simulink model "untitled"  (R2018b)
settings: Solver=VariableStepAuto  StartTime=0.0  StopTime=10.0  RelTol=1e-3
libraries: neural x29
settings Model: Creator=Paweł Tymiński  LastModifiedBy=Paweł Tymiński

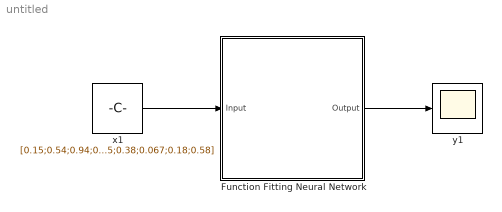
== system untitled ==
  Function Fitting Neural Network : Subsystem
      mask help: Function Fitting Neural Network
      mask Display: e = 0.06;c1 = [120 150 230]/255;c2 = ([120 150 230]+0)/383;c3 = ([120 150 230]+128)/383;patch([0 1 1 0],[0 0 1 1],c1);patch([0 1 1 1-e 1-e 0+e],[0 0 1 1-e 0+e 0+e],c2);patch([0 0 1 1-e 0+e 0+e],[0 1 1 1-e 1-e 0+e],c3);plot([0 1 1 0 0],[0 0 1 1 0]);fprintf('NNET');port_label('input',1,' Input');port_label('output',1,'Output ');
  x1 : Constant  Value=[0.15;0.54;0.94;0.66;0.39;0.26;0.85;0.95;0.38;0.067;0.18;0.58]  SampleTime=1
      mask Display: e = 0.06;c1 = [120 230 180]/255;c2 = ([120 230 180]+0)/(256+128);c3 = ([120 230 180]+128)/(256+128);patch([0 1 1 0],[0 0 1 1],c1);patch([0 1 1 1-e 1-e 0+e],[0 0 1 1-e 0+e 0+e],c2);patch([0 0 1 1-e 0+e 0+e],[0 1 1 1-e 1-e 0+e],c3);plot([0 1 1 0 0],[0 0 1 1 0]);disp('Constant');
  y1 : Scope
      mask Display: e = 0.06;c1 = [120 230 180]/255;c2 = ([120 230 180]+0)/(256+128);c3 = ([120 230 180]+128)/(256+128);patch([0 1 1 0],[0 0 1 1],c1);patch([0 1 1 1-e 1-e 0+e],[0 0 1 1-e 0+e 0+e],c2);patch([0 0 1 1-e 0+e 0+e],[0 1 1 1-e 1-e 0+e],c3);plot([0 1 1 0 0],[0 0 1 1 0]);plot([0.15 0.85 0.85 0.15 0.15],[0.5 0.5 0.85 0.85 0.5]);
  wires:
  x1/1 -> Function Fitting Neural Network/1(Input)
  Function Fitting Neural Network/1(Output) -> y1/1

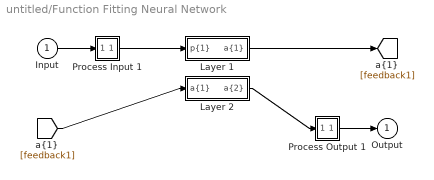
== system untitled/Function Fitting Neural Network ==
  Input : Inport  PortDimensions=12
      mask Display: e = 0.06;c1 = [120 230 180]/255;c2 = ([120 230 180]+0)/(256+128);c3 = ([120 230 180]+128)/(256+128);patch([0 1 1 0],[0 0 1 1],c1);patch([0 1 1 1-e 1-e 0+e],[0 0 1 1-e 0+e 0+e],c2);patch([0 0 1 1-e 0+e 0+e],[0 1 1 1-e 1-e 0+e],c3);plot([0 1 1 0 0],[0 0 1 1 0]);
  Layer 1 : Subsystem
      mask Display: e = 0.06;c1 = [120 150 230]/255;c2 = ([120 150 230]+0)/383;c3 = ([120 150 230]+128)/383;patch([0 1 1 0],[0 0 1 1],c1);patch([0 1 1 1-e 1-e 0+e],[0 0 1 1-e 0+e 0+e],c2);patch([0 0 1 1-e 0+e 0+e],[0 1 1 1-e 1-e 0+e],c3);plot([0 1 1 0 0],[0 0 1 1 0]);
  Layer 2 : Subsystem
      mask Display: e = 0.06;c1 = [120 150 230]/255;c2 = ([120 150 230]+0)/383;c3 = ([120 150 230]+128)/383;patch([0 1 1 0],[0 0 1 1],c1);patch([0 1 1 1-e 1-e 0+e],[0 0 1 1-e 0+e 0+e],c2);patch([0 0 1 1-e 0+e 0+e],[0 1 1 1-e 1-e 0+e],c3);plot([0 1 1 0 0],[0 0 1 1 0]);
  Process Input 1 : Subsystem
      mask Display: e = 0.06;c1 = [120 150 230]/255;c2 = ([120 150 230]+0)/383;c3 = ([120 150 230]+128)/383;patch([0 1 1 0],[0 0 1 1],c1);patch([0 1 1 1-e 1-e 0+e],[0 0 1 1-e 0+e 0+e],c2);patch([0 0 1 1-e 0+e 0+e],[0 1 1 1-e 1-e 0+e],c3);plot([0 1 1 0 0],[0 0 1 1 0]);
  Process Output 1 : Subsystem
      mask Display: e = 0.06;c1 = [120 150 230]/255;c2 = ([120 150 230]+0)/383;c3 = ([120 150 230]+128)/383;patch([0 1 1 0],[0 0 1 1],c1);patch([0 1 1 1-e 1-e 0+e],[0 0 1 1-e 0+e 0+e],c2);patch([0 0 1 1-e 0+e 0+e],[0 1 1 1-e 1-e 0+e],c3);plot([0 1 1 0 0],[0 0 1 1 0]);
  Output : Outport  InitialOutput=0
      mask Display: e = 0.06;c1 = [120 230 180]/255;c2 = ([120 230 180]+0)/(256+128);c3 = ([120 230 180]+128)/(256+128);patch([0 1 1 0],[0 0 1 1],c1);patch([0 1 1 1-e 1-e 0+e],[0 0 1 1-e 0+e 0+e],c2);patch([0 0 1 1-e 0+e 0+e],[0 1 1 1-e 1-e 0+e],c3);plot([0 1 1 0 0],[0 0 1 1 0]);
  wires:
  Input/1 -> Process Input 1/1(x)
  Process Output 1/1(y) -> Output/1
  Process Input 1/1(p) -> Layer 1/1("p{1}")
  Layer 1/1("a{1}") -> [feedback1]
  [feedback1] -> Layer 2/1("a{1} ")
  Layer 2/1("a{2}") -> Process Output 1/1(a)

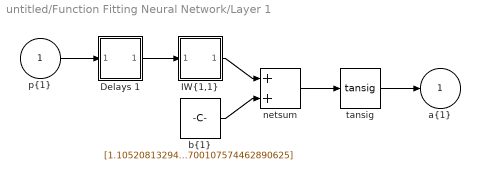
== system untitled/Function Fitting Neural Network/Layer 1 ==
  "p{1}" : Inport  PortDimensions=12
      mask Display: e = 0.06;c1 = [120 230 180]/255;c2 = ([120 230 180]+0)/(256+128);c3 = ([120 230 180]+128)/(256+128);patch([0 1 1 0],[0 0 1 1],c1);patch([0 1 1 1-e 1-e 0+e],[0 0 1 1-e 0+e 0+e],c2);patch([0 0 1 1-e 0+e 0+e],[0 1 1 1-e 1-e 0+e],c3);plot([0 1 1 0 0],[0 0 1 1 0]);
  Delays 1 : Subsystem
      mask Display: e = 0.06;c1 = [120 150 230]/255;c2 = ([120 150 230]+0)/383;c3 = ([120 150 230]+128)/383;patch([0 1 1 0],[0 0 1 1],c1);patch([0 1 1 1-e 1-e 0+e],[0 0 1 1-e 0+e 0+e],c2);patch([0 0 1 1-e 0+e 0+e],[0 1 1 1-e 1-e 0+e],c3);plot([0 1 1 0 0],[0 0 1 1 0]);disp('0');
  "IW{1,1}" : Subsystem
      mask Display: e = 0.06;c1 = [120 150 230]/255;c2 = ([120 150 230]+0)/383;c3 = ([120 150 230]+128)/383;patch([0 1 1 0],[0 0 1 1],c1);patch([0 1 1 1-e 1-e 0+e],[0 0 1 1-e 0+e 0+e],c2);patch([0 0 1 1-e 0+e 0+e],[0 1 1 1-e 1-e 0+e],c3);plot([0 1 1 0 0],[0 0 1 1 0]);disp('W');
  "b{1}" : Constant  Value=[1.105208132943532373104744692682288587093353271484375;0.396650909628887216040737939692917279899120330810546875;0.54239414591900725337580979612539522349834442138671875;0.2115757327206850835210616423864848911762237548828125;-0.4515141543103080579157904139719903469085693359375;0.61502574896100348222915954465861432254314422607421875;0.01756516716692051172099553468797239474952220916748046875;0.6012622440599362239055380996433086693286895751953125;-0.051598209526726834805998578303842805325984954833984375;0.1426075559304570139484980018096393905580043792724609375;-0.2304812660871213558788639375052298419177532196044921875;0.0678801928230618190074352469309815205633640289306640625;-0.1511582018231164281640843682907870970666408538818359375;-0.04926365002972421525129220754024572670459747314453125;0.108299861116097961843962593775358982384204864501953125;0.3436669062178363542869874436291866004467010498046875;-0.156260455829143996009378270173328928649425506591796875;0.69466705870215761375874308214406482875347137451171875;0.35182399411871634331561153885559178888797760009765625;1.013705487305092578509402301278896629810333251953125;-0.341177188449490298438604440889321267604827880859375;0.07182603963840873684265631027301424182951450347900390625;0.61566924743637507777549444654141552746295928955078125;-0.243279720160138490658852106207632459700107574462890625]
      mask Display: e = 0.06;c1 = [120 150 230]/255;c2 = ([120 150 230]+0)/383;c3 = ([120 150 230]+128)/383;patch([0 1 1 0],[0 0 1 1],c1);patch([0 1 1 1-e 1-e 0+e],[0 0 1 1-e 0+e 0+e],c2);patch([0 0 1 1-e 0+e 0+e],[0 1 1 1-e 1-e 0+e],c3);plot([0 1 1 0 0],[0 0 1 1 0]);disp('b');
  netsum : Sum  Inputs=2  SaturateOnIntegerOverflow=on  InputSameDT=on  OutDataTypeStr=Inherit: Same as first input
      mask Display: e = 0.06;c1 = [120 150 230]/255;c2 = ([120 150 230]+0)/383;c3 = ([120 150 230]+128)/383;patch([0 1 1 0],[0 0 1 1],c1);patch([0 1 1 1-e 1-e 0+e],[0 0 1 1-e 0+e 0+e],c2);patch([0 0 1 1-e 0+e 0+e],[0 1 1 1-e 1-e 0+e],c3);plot([0 1 1 0 0],[0 0 1 1 0]);disp('+');
  tansig : neural/Transfer Functions/tansig
  "a{1}" : Outport  InitialOutput=[0;0;0;0;0;0;0;0;0;0;0;0;0;0;0;0;0;0;0;0;0;0;0;0]
      mask Display: e = 0.06;c1 = [120 230 180]/255;c2 = ([120 230 180]+0)/(256+128);c3 = ([120 230 180]+128)/(256+128);patch([0 1 1 0],[0 0 1 1],c1);patch([0 1 1 1-e 1-e 0+e],[0 0 1 1-e 0+e 0+e],c2);patch([0 0 1 1-e 0+e 0+e],[0 1 1 1-e 1-e 0+e],c3);plot([0 1 1 0 0],[0 0 1 1 0]);
  wires:
  "p{1}"/1 -> Delays 1/1("p{1}")
  Delays 1/1("pd{1,1}") -> "IW{1,1}"/1("pd{1,1}")
  "IW{1,1}"/1("iz{1,1}") -> netsum/1
  "b{1}"/1 -> netsum/2
  netsum/1 -> tansig/1
  tansig/1 -> "a{1}"/1

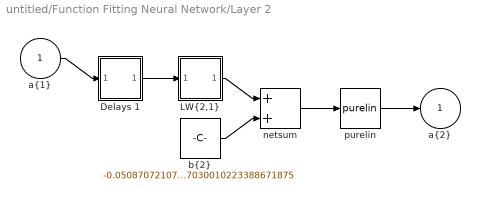
== system untitled/Function Fitting Neural Network/Layer 2 ==
  "a{1} " : Inport  PortDimensions=24
      mask Display: e = 0.06;c1 = [120 230 180]/255;c2 = ([120 230 180]+0)/(256+128);c3 = ([120 230 180]+128)/(256+128);patch([0 1 1 0],[0 0 1 1],c1);patch([0 1 1 1-e 1-e 0+e],[0 0 1 1-e 0+e 0+e],c2);patch([0 0 1 1-e 0+e 0+e],[0 1 1 1-e 1-e 0+e],c3);plot([0 1 1 0 0],[0 0 1 1 0]);
  Delays 1 : Subsystem
      mask Display: e = 0.06;c1 = [120 150 230]/255;c2 = ([120 150 230]+0)/383;c3 = ([120 150 230]+128)/383;patch([0 1 1 0],[0 0 1 1],c1);patch([0 1 1 1-e 1-e 0+e],[0 0 1 1-e 0+e 0+e],c2);patch([0 0 1 1-e 0+e 0+e],[0 1 1 1-e 1-e 0+e],c3);plot([0 1 1 0 0],[0 0 1 1 0]);disp('0');
  "LW{2,1}" : Subsystem
      mask Display: e = 0.06;c1 = [120 150 230]/255;c2 = ([120 150 230]+0)/383;c3 = ([120 150 230]+128)/383;patch([0 1 1 0],[0 0 1 1],c1);patch([0 1 1 1-e 1-e 0+e],[0 0 1 1-e 0+e 0+e],c2);patch([0 0 1 1-e 0+e 0+e],[0 1 1 1-e 1-e 0+e],c3);plot([0 1 1 0 0],[0 0 1 1 0]);disp('W');
  "b{2}" : Constant  Value=-0.050870721070801087904111881243807147257030010223388671875
      mask Display: e = 0.06;c1 = [120 150 230]/255;c2 = ([120 150 230]+0)/383;c3 = ([120 150 230]+128)/383;patch([0 1 1 0],[0 0 1 1],c1);patch([0 1 1 1-e 1-e 0+e],[0 0 1 1-e 0+e 0+e],c2);patch([0 0 1 1-e 0+e 0+e],[0 1 1 1-e 1-e 0+e],c3);plot([0 1 1 0 0],[0 0 1 1 0]);disp('b');
  netsum : Sum  Inputs=2  SaturateOnIntegerOverflow=on  InputSameDT=on  OutDataTypeStr=Inherit: Same as first input
      mask Display: e = 0.06;c1 = [120 150 230]/255;c2 = ([120 150 230]+0)/383;c3 = ([120 150 230]+128)/383;patch([0 1 1 0],[0 0 1 1],c1);patch([0 1 1 1-e 1-e 0+e],[0 0 1 1-e 0+e 0+e],c2);patch([0 0 1 1-e 0+e 0+e],[0 1 1 1-e 1-e 0+e],c3);plot([0 1 1 0 0],[0 0 1 1 0]);disp('+');
  purelin : neural/Transfer Functions/purelin
  "a{2}" : Outport  InitialOutput=0
      mask Display: e = 0.06;c1 = [120 230 180]/255;c2 = ([120 230 180]+0)/(256+128);c3 = ([120 230 180]+128)/(256+128);patch([0 1 1 0],[0 0 1 1],c1);patch([0 1 1 1-e 1-e 0+e],[0 0 1 1-e 0+e 0+e],c2);patch([0 0 1 1-e 0+e 0+e],[0 1 1 1-e 1-e 0+e],c3);plot([0 1 1 0 0],[0 0 1 1 0]);
  wires:
  "a{1} "/1 -> Delays 1/1("p{2}")
  Delays 1/1("pd{2,1}") -> "LW{2,1}"/1("ad{2,1}")
  "LW{2,1}"/1("lz{2,1}") -> netsum/1
  "b{2}"/1 -> netsum/2
  netsum/1 -> purelin/1
  purelin/1 -> "a{2}"/1

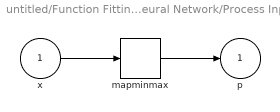
== system untitled/Function Fitting Neural Network/Process Input 1 ==
  x : Inport  PortDimensions=12
      mask Display: e = 0.06;c1 = [120 230 180]/255;c2 = ([120 230 180]+0)/(256+128);c3 = ([120 230 180]+128)/(256+128);patch([0 1 1 0],[0 0 1 1],c1);patch([0 1 1 1-e 1-e 0+e],[0 0 1 1-e 0+e 0+e],c2);patch([0 0 1 1-e 0+e 0+e],[0 1 1 1-e 1-e 0+e],c3);plot([0 1 1 0 0],[0 0 1 1 0]);
  mapminmax : neural/Processing Functions/mapminmax  xmin=[-3.14159265358979311599796346854;-3.14159265358979311599796346854;-3.14159265358979311599796346854;-3.14159265358979311599796346854;-3.14159265358979311599796346854;-3.14159265358979311599796346854;-3.14159265358979311599796346854;-3.14159265358979311599796346854;-3.14159265358979311599796346854;-3.14159265358979311599796346854;-3.14159265358979311599796346854;-3.14159265358979311599796346854]  xmax=[3.14159265358979311599796346854;3.14159265358979311599796346854;3.14159265358979311599796346854;3.14159265358979311599796346854;3.14159265358979311599796346854;3.14159265358979311599796346854;3.14159265358979311599796346854;3.14159265358979311599796346854;3.14159265358979311599796346854;3.14159265358979311599796346854;3.14159265358979311599796346854;3.14159265358979311599796346854]  ymin=-1  ymax=1
  p : Outport  PortDimensions=12
      mask Display: e = 0.06;c1 = [120 230 180]/255;c2 = ([120 230 180]+0)/(256+128);c3 = ([120 230 180]+128)/(256+128);patch([0 1 1 0],[0 0 1 1],c1);patch([0 1 1 1-e 1-e 0+e],[0 0 1 1-e 0+e 0+e],c2);patch([0 0 1 1-e 0+e 0+e],[0 1 1 1-e 1-e 0+e],c3);plot([0 1 1 0 0],[0 0 1 1 0]);
  wires:
  x/1 -> mapminmax/1
  mapminmax/1 -> p/1

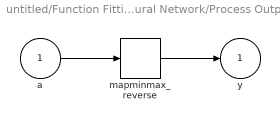
== system untitled/Function Fitting Neural Network/Process Output 1 ==
  a : Inport  PortDimensions=1
      mask Display: e = 0.06;c1 = [120 230 180]/255;c2 = ([120 230 180]+0)/(256+128);c3 = ([120 230 180]+128)/(256+128);patch([0 1 1 0],[0 0 1 1],c1);patch([0 1 1 1-e 1-e 0+e],[0 0 1 1-e 0+e 0+e],c2);patch([0 0 1 1-e 0+e 0+e],[0 1 1 1-e 1-e 0+e],c3);plot([0 1 1 0 0],[0 0 1 1 0]);
  mapminmax_reverse : neural/Processing Functions/mapminmax_reverse  xmin=-0.246707831183186704349097340128  xmax=0.224645518642549779642081375641  ymin=-1  ymax=1
  y : Outport  PortDimensions=1
      mask Display: e = 0.06;c1 = [120 230 180]/255;c2 = ([120 230 180]+0)/(256+128);c3 = ([120 230 180]+128)/(256+128);patch([0 1 1 0],[0 0 1 1],c1);patch([0 1 1 1-e 1-e 0+e],[0 0 1 1-e 0+e 0+e],c2);patch([0 0 1 1-e 0+e 0+e],[0 1 1 1-e 1-e 0+e],c3);plot([0 1 1 0 0],[0 0 1 1 0]);
  wires:
  a/1 -> mapminmax_reverse/1
  mapminmax_reverse/1 -> y/1

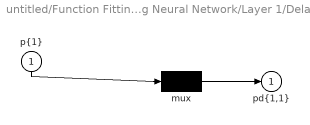
== system untitled/Function Fitting Neural Network/Layer 1/Delays 1 ==
  "p{1}" : Inport  PortDimensions=12
      mask Display: e = 0.06;c1 = [120 230 180]/255;c2 = ([120 230 180]+0)/(256+128);c3 = ([120 230 180]+128)/(256+128);patch([0 1 1 0],[0 0 1 1],c1);patch([0 1 1 1-e 1-e 0+e],[0 0 1 1-e 0+e 0+e],c2);patch([0 0 1 1-e 0+e 0+e],[0 1 1 1-e 1-e 0+e],c3);plot([0 1 1 0 0],[0 0 1 1 0]);
  mux : Mux  Inputs=1
      mask Display: e = 0.06;c1 = [120 150 230]/255;c2 = ([120 150 230]+0)/383;c3 = ([120 150 230]+128)/383;patch([0 1 1 0],[0 0 1 1],c1);patch([0 1 1 1-e 1-e 0+e],[0 0 1 1-e 0+e 0+e],c2);patch([0 0 1 1-e 0+e 0+e],[0 1 1 1-e 1-e 0+e],c3);plot([0 1 1 0 0],[0 0 1 1 0]);disp('Mux')
  "pd{1,1}" : Outport
      mask Display: e = 0.06;c1 = [120 230 180]/255;c2 = ([120 230 180]+0)/(256+128);c3 = ([120 230 180]+128)/(256+128);patch([0 1 1 0],[0 0 1 1],c1);patch([0 1 1 1-e 1-e 0+e],[0 0 1 1-e 0+e 0+e],c2);patch([0 0 1 1-e 0+e 0+e],[0 1 1 1-e 1-e 0+e],c3);plot([0 1 1 0 0],[0 0 1 1 0]);
  wires:
  "p{1}"/1 -> mux/1
  mux/1 -> "pd{1,1}"/1

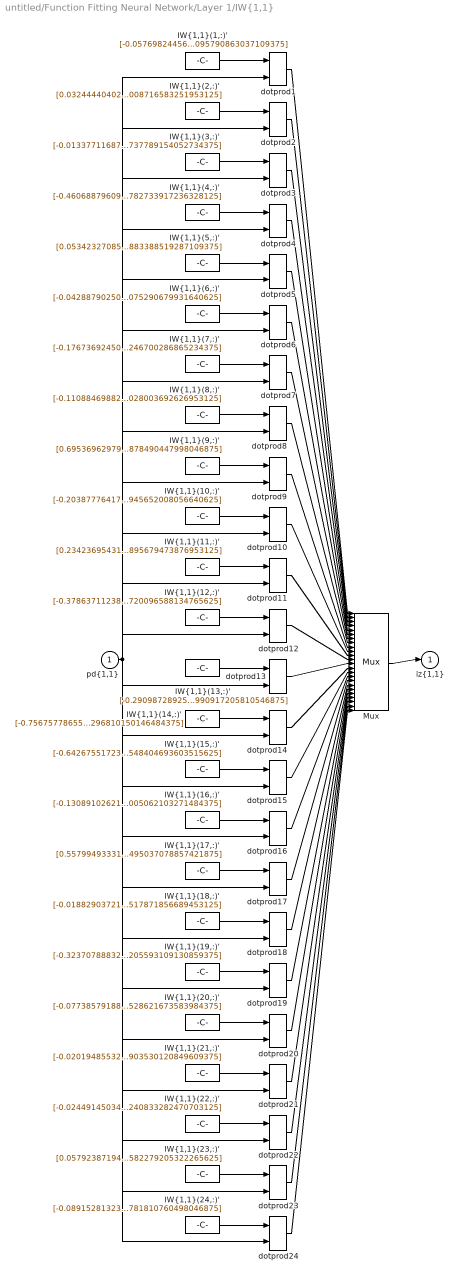
== system untitled/Function Fitting Neural Network/Layer 1/IW{1,1} ==
  "pd{1,1}" : Inport  PortDimensions=12
      mask Display: e = 0.06;c1 = [120 230 180]/255;c2 = ([120 230 180]+0)/(256+128);c3 = ([120 230 180]+128)/(256+128);patch([0 1 1 0],[0 0 1 1],c1);patch([0 1 1 1-e 1-e 0+e],[0 0 1 1-e 0+e 0+e],c2);patch([0 0 1 1-e 0+e 0+e],[0 1 1 1-e 1-e 0+e],c3);plot([0 1 1 0 0],[0 0 1 1 0]);
  "IW{1,1}(1,:)'" : Constant  Value=[-0.0576982445657482634349122463390813209116458892822265625;0.109430497477228716451946866072830744087696075439453125;-0.057052816673429408711459842606927850283682346343994140625;-0.00556308798543494499588835111580920056439936161041259765625;-0.6259020264135053412957176988129504024982452392578125;0.016003567569307701468073190653740311972796916961669921875;-0.8434917592845418976565952107193879783153533935546875;-0.82946259040420156072315194251132197678089141845703125;0.1764068613029800836056182333777542226016521453857421875;0.145967761274977736452029830616083927452564239501953125;-0.058731224497028937381326585409624385647475719451904296875;-0.81088898160597400188720484948134981095790863037109375]
      mask Display: e = 0.06;c1 = [120 150 230]/255;c2 = ([120 150 230]+0)/383;c3 = ([120 150 230]+128)/383;patch([0 1 1 0],[0 0 1 1],c1);patch([0 1 1 1-e 1-e 0+e],[0 0 1 1-e 0+e 0+e],c2);patch([0 0 1 1-e 0+e 0+e],[0 1 1 1-e 1-e 0+e],c3);plot([0 1 1 0 0],[0 0 1 1 0]);disp('Weights');
  "IW{1,1}(10,:)'" : Constant  Value=[-0.2038777641723933109485500381197198294103145599365234375;-0.09127744128260480149794631188342464156448841094970703125;-0.250425668125327349766706674927263520658016204833984375;-0.6005356078893466786894350661896169185638427734375;0.463817738348928643166146912335534580051898956298828125;-0.22254593099828123836658733125659637153148651123046875;0.58826545020638132399426467600278556346893310546875;0.44769782814802205894721964796190150082111358642578125;-0.62152830059035946153045415485394187271595001220703125;0.002081110896482388054884449246628719265572726726531982421875;-0.1693741871775031049285331619103089906275272369384765625;0.432919576819769391651249179631122387945652008056640625]
      mask Display: e = 0.06;c1 = [120 150 230]/255;c2 = ([120 150 230]+0)/383;c3 = ([120 150 230]+128)/383;patch([0 1 1 0],[0 0 1 1],c1);patch([0 1 1 1-e 1-e 0+e],[0 0 1 1-e 0+e 0+e],c2);patch([0 0 1 1-e 0+e 0+e],[0 1 1 1-e 1-e 0+e],c3);plot([0 1 1 0 0],[0 0 1 1 0]);disp('Weights');
  "IW{1,1}(11,:)'" : Constant  Value=[0.234236954316088319405508855197695083916187286376953125;-0.18360567694735241417447468847967684268951416015625;0.29527725169132512661462897085584700107574462890625;-0.07852522350352102165071954686936805956065654754638671875;-0.02499587978778217145503504070802591741085052490234375;0.55075537422061227044167708299937658011913299560546875;0.404000823445536727529514564594137482345104217529296875;0.44417301193162372907607959859888069331645965576171875;-0.098084331859639439787912351675913669168949127197265625;0.1552805895459416218873371917652548290789127349853515625;-0.105223174288441023715989786069258116185665130615234375;0.0273825467705861858025429000917938537895679473876953125]
      mask Display: e = 0.06;c1 = [120 150 230]/255;c2 = ([120 150 230]+0)/383;c3 = ([120 150 230]+128)/383;patch([0 1 1 0],[0 0 1 1],c1);patch([0 1 1 1-e 1-e 0+e],[0 0 1 1-e 0+e 0+e],c2);patch([0 0 1 1-e 0+e 0+e],[0 1 1 1-e 1-e 0+e],c3);plot([0 1 1 0 0],[0 0 1 1 0]);disp('Weights');
  "IW{1,1}(12,:)'" : Constant  Value=[-0.378637112386513818851341284243972040712833404541015625;0.037594262190869316697661162152144243009388446807861328125;-0.34276628323199143100197261446737684309482574462890625;0.5610059674731131540426076753647066652774810791015625;-0.234742924109086203987573071572114713490009307861328125;-0.34498433455168420191938594143721275031566619873046875;-0.40093355732895552545613782058353535830974578857421875;-0.244379228588640196040415730749373324215412139892578125;-0.2081185533989977354263345432627829723060131072998046875;-0.303788026176015024670817865626304410398006439208984375;0.497969472273695590303077551652677357196807861328125;-0.1530896961062103989181792940144077874720096588134765625]
      mask Display: e = 0.06;c1 = [120 150 230]/255;c2 = ([120 150 230]+0)/383;c3 = ([120 150 230]+128)/383;patch([0 1 1 0],[0 0 1 1],c1);patch([0 1 1 1-e 1-e 0+e],[0 0 1 1-e 0+e 0+e],c2);patch([0 0 1 1-e 0+e 0+e],[0 1 1 1-e 1-e 0+e],c3);plot([0 1 1 0 0],[0 0 1 1 0]);disp('Weights');
  "IW{1,1}(13,:)'" : Constant  Value=[-0.29098728925777483933501343926764093339443206787109375;-0.23403889436192637507616609582328237593173980712890625;-0.32648452880923806151969301936333067715167999267578125;0.37033303451168120279390905125183053314685821533203125;0.35741048081226012289590698856045491993427276611328125;-0.450714597452358589624310525323380716145038604736328125;-0.3935563897871983130016815266571938991546630859375;-0.169607468869786448539827006243285723030567169189453125;0.03627189488180206089484869380612508393824100494384765625;-0.255262783153725136831013742266804911196231842041015625;0.5406240190514794985432445173501037061214447021484375;0.3912157641259550455714588679256848990917205810546875]
      mask Display: e = 0.06;c1 = [120 150 230]/255;c2 = ([120 150 230]+0)/383;c3 = ([120 150 230]+128)/383;patch([0 1 1 0],[0 0 1 1],c1);patch([0 1 1 1-e 1-e 0+e],[0 0 1 1-e 0+e 0+e],c2);patch([0 0 1 1-e 0+e 0+e],[0 1 1 1-e 1-e 0+e],c3);plot([0 1 1 0 0],[0 0 1 1 0]);disp('Weights');
  "IW{1,1}(14,:)'" : Constant  Value=[-0.75675778655779823989036003695218823850154876708984375;-0.57256728570934745103926388765103183686733245849609375;-0.69813783058899481215320292903925292193889617919921875;0.341299029411496090968825001255027018487453460693359375;0.251303173023257497842308794133714400231838226318359375;-0.404678403021913657422459209556109271943569183349609375;-0.46178764454366716396549463752307929098606109619140625;-0.612694179813959127756106681772507727146148681640625;-0.1787251079729085534442134530763723887503147125244140625;-0.0708295086322307809734155625847051851451396942138671875;0.28467844523556140590159202474751509726047515869140625;0.253402445405866261207705747438012622296810150146484375]
      mask Display: e = 0.06;c1 = [120 150 230]/255;c2 = ([120 150 230]+0)/383;c3 = ([120 150 230]+128)/383;patch([0 1 1 0],[0 0 1 1],c1);patch([0 1 1 1-e 1-e 0+e],[0 0 1 1-e 0+e 0+e],c2);patch([0 0 1 1-e 0+e 0+e],[0 1 1 1-e 1-e 0+e],c3);plot([0 1 1 0 0],[0 0 1 1 0]);disp('Weights');
  "IW{1,1}(15,:)'" : Constant  Value=[-0.642675517239493121479654291761107742786407470703125;0.454770625971706754508971926043159328401088714599609375;-0.55909130185978284099945767593453638255596160888671875;-0.324232449901053210172818808132433332502841949462890625;-0.3021864416171464728932960497331805527210235595703125;0.025746204309359012329938565244447090663015842437744140625;0.29076344251290031639456401535426266491413116455078125;0.287224819587555690869606905835098586976528167724609375;0.5660394222826548027427406850620172917842864990234375;0.59714965990429702547004353618831373751163482666015625;0.1381454207647970500172363017554744146764278411865234375;-0.1817547750427616348734005669030011631548404693603515625]
      mask Display: e = 0.06;c1 = [120 150 230]/255;c2 = ([120 150 230]+0)/383;c3 = ([120 150 230]+128)/383;patch([0 1 1 0],[0 0 1 1],c1);patch([0 1 1 1-e 1-e 0+e],[0 0 1 1-e 0+e 0+e],c2);patch([0 0 1 1-e 0+e 0+e],[0 1 1 1-e 1-e 0+e],c3);plot([0 1 1 0 0],[0 0 1 1 0]);disp('Weights');
  "IW{1,1}(16,:)'" : Constant  Value=[-0.130891026211613858976079427520744502544403076171875;0.66844103513181496456496688551851548254489898681640625;-0.077856732269279138591855371487326920032501220703125;-0.232472090221449156910438205159152857959270477294921875;-0.255710980073264926293319376782164908945560455322265625;-0.4776360697880968064765738745336420834064483642578125;-0.43032739202462166883123018124024383723735809326171875;-0.315093839860602853431004177764407359063625335693359375;0.42425139290134550318356332354596816003322601318359375;0.1627815184339168330662772632422274909913539886474609375;-0.175561382573102442439250125971739180386066436767578125;-0.195398308804458353815647342344163917005062103271484375]
      mask Display: e = 0.06;c1 = [120 150 230]/255;c2 = ([120 150 230]+0)/383;c3 = ([120 150 230]+128)/383;patch([0 1 1 0],[0 0 1 1],c1);patch([0 1 1 1-e 1-e 0+e],[0 0 1 1-e 0+e 0+e],c2);patch([0 0 1 1-e 0+e 0+e],[0 1 1 1-e 1-e 0+e],c3);plot([0 1 1 0 0],[0 0 1 1 0]);disp('Weights');
  "IW{1,1}(17,:)'" : Constant  Value=[0.55799493331606042634263076251954771578311920166015625;-0.22309655693261698505835965988808311522006988525390625;0.6126227320923636199268003110773861408233642578125;0.58402488695494059189883273575105704367160797119140625;0.0611459190998968338259800248124520294368267059326171875;-0.1009568503039272313603902375689358450472354888916015625;-0.0027857496668865773352397052775586416828446090221405029296875;-0.043533707626254448952440867515178979374468326568603515625;-0.423914476654462302196435530277085490524768829345703125;-0.297306405257678652009900588382151909172534942626953125;0.31034488341500965358221719725406728684902191162109375;0.138219760650011458391617225061054341495037078857421875]
      mask Display: e = 0.06;c1 = [120 150 230]/255;c2 = ([120 150 230]+0)/383;c3 = ([120 150 230]+128)/383;patch([0 1 1 0],[0 0 1 1],c1);patch([0 1 1 1-e 1-e 0+e],[0 0 1 1-e 0+e 0+e],c2);patch([0 0 1 1-e 0+e 0+e],[0 1 1 1-e 1-e 0+e],c3);plot([0 1 1 0 0],[0 0 1 1 0]);disp('Weights');
  "IW{1,1}(18,:)'" : Constant  Value=[-0.0188290372159080586500490284151965170167386531829833984375;0.08571894067923425952759686197168775834143161773681640625;0.07476998276994810399553870183808612637221813201904296875;-0.26273279809814109597709830268286168575286865234375;0.74529773641065133471528270092676393687725067138671875;0.2287956900511584346080695695491158403456211090087890625;0.100676777302572684202885966442408971488475799560546875;0.10545777470751178939156744718275149352848529815673828125;-0.33779422396237623882342404613154940307140350341796875;-0.10004153793748025991217076580142020247876644134521484375;-0.314650660060184328425947342111612670123577117919921875;0.717674975622703659183798663434572517871856689453125]
      mask Display: e = 0.06;c1 = [120 150 230]/255;c2 = ([120 150 230]+0)/383;c3 = ([120 150 230]+128)/383;patch([0 1 1 0],[0 0 1 1],c1);patch([0 1 1 1-e 1-e 0+e],[0 0 1 1-e 0+e 0+e],c2);patch([0 0 1 1-e 0+e 0+e],[0 1 1 1-e 1-e 0+e],c3);plot([0 1 1 0 0],[0 0 1 1 0]);disp('Weights');
  "IW{1,1}(19,:)'" : Constant  Value=[-0.323707888322097014910383450114750303328037261962890625;-0.1829168855639349555719519457852584309875965118408203125;-0.330005694199064947280675141882966272532939910888671875;-0.731949829581310940085359106888063251972198486328125;-0.08612571232734229920158242066463571973145008087158203125;-0.08059809728553703200848445931114838458597660064697265625;-0.87760323631197678651005844585597515106201171875;-0.80758494986182449704159580505802296102046966552734375;-0.60381485601594520051804693139274604618549346923828125;-0.094564858083827363355311490522581152617931365966796875;-0.1287633543330141960847612381257931701838970184326171875;-0.184875298135876331429017227492295205593109130859375]
      mask Display: e = 0.06;c1 = [120 150 230]/255;c2 = ([120 150 230]+0)/383;c3 = ([120 150 230]+128)/383;patch([0 1 1 0],[0 0 1 1],c1);patch([0 1 1 1-e 1-e 0+e],[0 0 1 1-e 0+e 0+e],c2);patch([0 0 1 1-e 0+e 0+e],[0 1 1 1-e 1-e 0+e],c3);plot([0 1 1 0 0],[0 0 1 1 0]);disp('Weights');
  "IW{1,1}(2,:)'" : Constant  Value=[0.032444404023012941851167312279358156956732273101806640625;0.04414553061315297510791566537591279484331607818603515625;-0.0106112782487167885137058220834660460241138935089111328125;-0.048784886253699526192928459522590856067836284637451171875;0.2277580941245788415105977264829562045633792877197265625;-0.033054502953275687049394804262192337773740291595458984375;-0.227154873776603649648819782669306732714176177978515625;-0.280258960188446260008987565015559084713459014892578125;0.042431749134326561534447108670065063051879405975341796875;0.02391057263545350031197500584312365390360355377197265625;0.56944118083220163217816889300593174993991851806640625;0.228972666740030750265333381321397610008716583251953125]
      mask Display: e = 0.06;c1 = [120 150 230]/255;c2 = ([120 150 230]+0)/383;c3 = ([120 150 230]+128)/383;patch([0 1 1 0],[0 0 1 1],c1);patch([0 1 1 1-e 1-e 0+e],[0 0 1 1-e 0+e 0+e],c2);patch([0 0 1 1-e 0+e 0+e],[0 1 1 1-e 1-e 0+e],c3);plot([0 1 1 0 0],[0 0 1 1 0]);disp('Weights');
  "IW{1,1}(20,:)'" : Constant  Value=[-0.077385791888315680342458335871924646198749542236328125;-0.07791169269795907015296876352294930256903171539306640625;-0.1197486847395914655312054719615844078361988067626953125;0.01236999838006685135949336284966193488799035549163818359375;-0.12042939319783500795590924781208741478621959686279296875;0.1777993058522819025402128545465529896318912506103515625;1.256154726931602905182217000401578843593597412109375;1.1044308939133369307228349498473107814788818359375;-0.06957830754075521040302731989868334494531154632568359375;0.06102650058959908918598813443168182857334613800048828125;0.1265492084764261171425658858424867503345012664794921875;-0.12455408350473749778952736733117490075528621673583984375]
      mask Display: e = 0.06;c1 = [120 150 230]/255;c2 = ([120 150 230]+0)/383;c3 = ([120 150 230]+128)/383;patch([0 1 1 0],[0 0 1 1],c1);patch([0 1 1 1-e 1-e 0+e],[0 0 1 1-e 0+e 0+e],c2);patch([0 0 1 1-e 0+e 0+e],[0 1 1 1-e 1-e 0+e],c3);plot([0 1 1 0 0],[0 0 1 1 0]);disp('Weights');
  "IW{1,1}(21,:)'" : Constant  Value=[-0.0201948553262207806946459953678640886209905147552490234375;-0.23862416360800586812018764248932711780071258544921875;-0.0624075719155085806288951744136284105479717254638671875;-0.2050412304881187586236279685181216336786746978759765625;0.57755863849575195256846882330137304961681365966796875;-0.1868015885482841864639880213871947489678859710693359375;-1.1297969667168483720587346397223882377147674560546875;-1.0499418410353704711468481036718003451824188232421875;0.11028483750953076147904852177816792391240596771240234375;-0.01477289766724391821550721459743726882152259349822998046875;-0.36103070488242094970843254486680962145328521728515625;0.490549489427872520419526836121804080903530120849609375]
      mask Display: e = 0.06;c1 = [120 150 230]/255;c2 = ([120 150 230]+0)/383;c3 = ([120 150 230]+128)/383;patch([0 1 1 0],[0 0 1 1],c1);patch([0 1 1 1-e 1-e 0+e],[0 0 1 1-e 0+e 0+e],c2);patch([0 0 1 1-e 0+e 0+e],[0 1 1 1-e 1-e 0+e],c3);plot([0 1 1 0 0],[0 0 1 1 0]);disp('Weights');
  "IW{1,1}(22,:)'" : Constant  Value=[-0.0244914503415263780372601587487224605865776538848876953125;-0.364372965754643729496820014901459217071533203125;0.0243159411388128264552843660339931375347077846527099609375;-0.37098362235615400805954777752049267292022705078125;-0.4495515370744975758299233348225243389606475830078125;-0.136068426983480039726970289848395623266696929931640625;0.93762933653948088430496454748208634555339813232421875;0.90477946186466839950668372694053687155246734619140625;-0.03000179655139802170626950328369275666773319244384765625;-0.02314507042774012479657841367952642031013965606689453125;-0.3708231204690406457302742637693881988525390625;-0.459923018655834792145498113313806243240833282470703125]
      mask Display: e = 0.06;c1 = [120 150 230]/255;c2 = ([120 150 230]+0)/383;c3 = ([120 150 230]+128)/383;patch([0 1 1 0],[0 0 1 1],c1);patch([0 1 1 1-e 1-e 0+e],[0 0 1 1-e 0+e 0+e],c2);patch([0 0 1 1-e 0+e 0+e],[0 1 1 1-e 1-e 0+e],c3);plot([0 1 1 0 0],[0 0 1 1 0]);disp('Weights');
  "IW{1,1}(23,:)'" : Constant  Value=[0.057923871941129724538743772654925123788416385650634765625;-0.038101758688630339710901040461976663209497928619384765625;-0.056767019092911215338848052169851143844425678253173828125;-0.1377024091174046116492490909877233207225799560546875;0.6678687518898216435303538673906587064266204833984375;0.016842694778476163808278442957089282572269439697265625;-0.573627643756173366540451752371154725551605224609375;-0.54305860239335956851647324583609588444232940673828125;-0.2162603534989049058889776233627344481647014617919921875;-0.0307499419002988071125681557305142632685601711273193359375;-0.351361160413071027530662604476674459874629974365234375;0.68426041126203307474185066894278861582279205322265625]
      mask Display: e = 0.06;c1 = [120 150 230]/255;c2 = ([120 150 230]+0)/383;c3 = ([120 150 230]+128)/383;patch([0 1 1 0],[0 0 1 1],c1);patch([0 1 1 1-e 1-e 0+e],[0 0 1 1-e 0+e 0+e],c2);patch([0 0 1 1-e 0+e 0+e],[0 1 1 1-e 1-e 0+e],c3);plot([0 1 1 0 0],[0 0 1 1 0]);disp('Weights');
  "IW{1,1}(24,:)'" : Constant  Value=[-0.089152813230756577933533435498247854411602020263671875;-0.262769720128436912176539408392272889614105224609375;-0.10479759655914454297143123540081433020532131195068359375;0.1345656369837241739251254557530046440660953521728515625;0.40740216246193072802128654075204394757747650146484375;-0.2194822663390892103496554454977740533649921417236328125;0.356598886658677172167841717964620329439640045166015625;0.1702564951638410317702465590627980418503284454345703125;0.17709175951611733079715804706211201846599578857421875;-0.252332025293368344964761718074441887438297271728515625;-0.382111621215373953308613863555365242063999176025390625;0.251446899431794601564860158759984187781810760498046875]
      mask Display: e = 0.06;c1 = [120 150 230]/255;c2 = ([120 150 230]+0)/383;c3 = ([120 150 230]+128)/383;patch([0 1 1 0],[0 0 1 1],c1);patch([0 1 1 1-e 1-e 0+e],[0 0 1 1-e 0+e 0+e],c2);patch([0 0 1 1-e 0+e 0+e],[0 1 1 1-e 1-e 0+e],c3);plot([0 1 1 0 0],[0 0 1 1 0]);disp('Weights');
  "IW{1,1}(3,:)'" : Constant  Value=[-0.0133771168748701395345701570249730139039456844329833984375;0.0763063424342609319950270219123922288417816162109375;-0.00433239973336086749144957508406150736846029758453369140625;-0.26987809520125549678226661853841505944728851318359375;-0.57059338983247098742168645912897773087024688720703125;0.384368842152972789438791778593440540134906768798828125;-0.1256256707437911346314507454735576175153255462646484375;-0.0685123040543063333007722803813521750271320343017578125;0.08779416068995703203992064800331718288362026214599609375;0.09337886326118394197948191504110582172870635986328125;-0.58740380496223909556618991700815968215465545654296875;-0.478799230213843907133508537299348972737789154052734375]
      mask Display: e = 0.06;c1 = [120 150 230]/255;c2 = ([120 150 230]+0)/383;c3 = ([120 150 230]+128)/383;patch([0 1 1 0],[0 0 1 1],c1);patch([0 1 1 1-e 1-e 0+e],[0 0 1 1-e 0+e 0+e],c2);patch([0 0 1 1-e 0+e 0+e],[0 1 1 1-e 1-e 0+e],c3);plot([0 1 1 0 0],[0 0 1 1 0]);disp('Weights');
  "IW{1,1}(4,:)'" : Constant  Value=[-0.460688796099610053946804555380367673933506011962890625;0.0218327475783109577200935547125482116825878620147705078125;-0.41820654442267091166485215580905787646770477294921875;-0.4904504828200233479407188497134484350681304931640625;0.2167308489218358336092506988279637880623340606689453125;-0.504435540456765973971187122515402734279632568359375;-0.07280012887168653412661711854525492526590824127197265625;-0.0208240398345085619968841683657956309616565704345703125;-0.49580671789337082966397929340018890798091888427734375;0.1516105008590765412801459888214594684541225433349609375;-0.01210911724616351749228559953053263598121702671051025390625;0.21213081019141555305651536400546319782733917236328125]
      mask Display: e = 0.06;c1 = [120 150 230]/255;c2 = ([120 150 230]+0)/383;c3 = ([120 150 230]+128)/383;patch([0 1 1 0],[0 0 1 1],c1);patch([0 1 1 1-e 1-e 0+e],[0 0 1 1-e 0+e 0+e],c2);patch([0 0 1 1-e 0+e 0+e],[0 1 1 1-e 1-e 0+e],c3);plot([0 1 1 0 0],[0 0 1 1 0]);disp('Weights');
  "IW{1,1}(5,:)'" : Constant  Value=[0.0534232708597609795564409296275698579847812652587890625;0.16774363146205051311454781171050854027271270751953125;0.0557262696741866181415758774164714850485324859619140625;0.149943034202409897215346745724673382937908172607421875;-0.7583570447809131476191168985678814351558685302734375;0.021572203247338793408172108456710702739655971527099609375;-1.311766860438324133752985289902426302433013916015625;-1.3538622540610190103649301818222738802433013916015625;0.2321862915409871053196155799014377407729625701904296875;0.021289639636092684560342291888446197845041751861572265625;0.0007997458642366793261924140523433379712514579296112060546875;-0.7273831484000989888727417564950883388519287109375]
      mask Display: e = 0.06;c1 = [120 150 230]/255;c2 = ([120 150 230]+0)/383;c3 = ([120 150 230]+128)/383;patch([0 1 1 0],[0 0 1 1],c1);patch([0 1 1 1-e 1-e 0+e],[0 0 1 1-e 0+e 0+e],c2);patch([0 0 1 1-e 0+e 0+e],[0 1 1 1-e 1-e 0+e],c3);plot([0 1 1 0 0],[0 0 1 1 0]);disp('Weights');
  "IW{1,1}(6,:)'" : Constant  Value=[-0.042887902504551482507633153318238328211009502410888671875;0.10011698198800951520315294374086079187691211700439453125;0.0183947098946129240781832692164243781007826328277587890625;0.0183753700627734863071172100035255425609648227691650390625;0.8318443763359837372917127140681259334087371826171875;-0.06148931737005235154125415419912314973771572113037109375;-1.43741329717547738908933752099983394145965576171875;-1.344111704553765829217581995180808007717132568359375;-0.002083691936784548733030408840249947388656437397003173828125;0.0219070192460075474638614423383842222392559051513671875;-0.1227729899922761214181576860937639139592647552490234375;0.757250047484776533934791586943902075290679931640625]
      mask Display: e = 0.06;c1 = [120 150 230]/255;c2 = ([120 150 230]+0)/383;c3 = ([120 150 230]+128)/383;patch([0 1 1 0],[0 0 1 1],c1);patch([0 1 1 1-e 1-e 0+e],[0 0 1 1-e 0+e 0+e],c2);patch([0 0 1 1-e 0+e 0+e],[0 1 1 1-e 1-e 0+e],c3);plot([0 1 1 0 0],[0 0 1 1 0]);disp('Weights');
  "IW{1,1}(7,:)'" : Constant  Value=[-0.1767369245088252771580528133199550211429595947265625;0.5846053848789203311042683708365075290203094482421875;-0.30133591823106986584690503150341100990772247314453125;0.1189048734166412712998095457805902697145938873291015625;-0.271097225218794923851106659640208818018436431884765625;-0.07763389618348419396465232011905754916369915008544921875;0.1905032244730675283772569628126802854239940643310546875;0.24022728040993468479058492448530159890651702880859375;0.09425656956632884331259703003524919040501117706298828125;0.2230703627708460479173169233035878278315067291259765625;0.354585433082117262859611628300626762211322784423828125;-0.4509166883292985428255406077369116246700286865234375]
      mask Display: e = 0.06;c1 = [120 150 230]/255;c2 = ([120 150 230]+0)/383;c3 = ([120 150 230]+128)/383;patch([0 1 1 0],[0 0 1 1],c1);patch([0 1 1 1-e 1-e 0+e],[0 0 1 1-e 0+e 0+e],c2);patch([0 0 1 1-e 0+e 0+e],[0 1 1 1-e 1-e 0+e],c3);plot([0 1 1 0 0],[0 0 1 1 0]);disp('Weights');
  "IW{1,1}(8,:)'" : Constant  Value=[-0.1108846988293971935757298297176021151244640350341796875;-0.10516689556990044263073968977550975978374481201171875;-0.1174807690235275814405468963741441257297992706298828125;-0.27720500943029391383021220462978817522525787353515625;-0.64176101470788593506000552224577404558658599853515625;-0.198343832944798348361103990100673399865627288818359375;-1.3164808274923698316882791914395056664943695068359375;-1.200746314138724901710020276368595659732818603515625;-0.1532839083486366715813886685282341204583644866943359375;-0.0884209303619780673244576973957009613513946533203125;-0.0019793400072741613136828586760884718387387692928314208984375;-0.44963244460985951622689071882632561028003692626953125]
      mask Display: e = 0.06;c1 = [120 150 230]/255;c2 = ([120 150 230]+0)/383;c3 = ([120 150 230]+128)/383;patch([0 1 1 0],[0 0 1 1],c1);patch([0 1 1 1-e 1-e 0+e],[0 0 1 1-e 0+e 0+e],c2);patch([0 0 1 1-e 0+e 0+e],[0 1 1 1-e 1-e 0+e],c3);plot([0 1 1 0 0],[0 0 1 1 0]);disp('Weights');
  "IW{1,1}(9,:)'" : Constant  Value=[0.69536962979951855157167983634280972182750701904296875;0.313437225800806296138745210555498488247394561767578125;0.70548615420570592871030157766654156148433685302734375;0.36918947301072735367455379673629067838191986083984375;-0.15588613080115465425734555537928827106952667236328125;0.086186720057942978190368421564926393330097198486328125;0.5683638702513060803056532677146606147289276123046875;0.362798348076213639235021446438622660934925079345703125;-0.0408971182268364208400868164972052909433841705322265625;-0.0552198065087323997079948867394705303013324737548828125;0.421265198246681571436766944316332228481769561767578125;-0.1500073563638377460716100131321582011878490447998046875]
      mask Display: e = 0.06;c1 = [120 150 230]/255;c2 = ([120 150 230]+0)/383;c3 = ([120 150 230]+128)/383;patch([0 1 1 0],[0 0 1 1],c1);patch([0 1 1 1-e 1-e 0+e],[0 0 1 1-e 0+e 0+e],c2);patch([0 0 1 1-e 0+e 0+e],[0 1 1 1-e 1-e 0+e],c3);plot([0 1 1 0 0],[0 0 1 1 0]);disp('Weights');
  Mux : Mux  Inputs=24
      mask Display: e = 0.06;c1 = [120 150 230]/255;c2 = ([120 150 230]+0)/383;c3 = ([120 150 230]+128)/383;patch([0 1 1 0],[0 0 1 1],c1);patch([0 1 1 1-e 1-e 0+e],[0 0 1 1-e 0+e 0+e],c2);patch([0 0 1 1-e 0+e 0+e],[0 1 1 1-e 1-e 0+e],c3);plot([0 1 1 0 0],[0 0 1 1 0]);disp('Mux');
  dotprod{1..24} (24 alike) : neural/Weight Functions/dotprod
  "iz{1,1}" : Outport
      mask Display: e = 0.06;c1 = [120 230 180]/255;c2 = ([120 230 180]+0)/(256+128);c3 = ([120 230 180]+128)/(256+128);patch([0 1 1 0],[0 0 1 1],c1);patch([0 1 1 1-e 1-e 0+e],[0 0 1 1-e 0+e 0+e],c2);patch([0 0 1 1-e 0+e 0+e],[0 1 1 1-e 1-e 0+e],c3);plot([0 1 1 0 0],[0 0 1 1 0]);
  wires:
  "IW{1,1}(1,:)'"/1 -> dotprod1/1
  "pd{1,1}"/1 -> dotprod1/2, dotprod2/2, dotprod3/2, dotprod4/2, dotprod5/2, dotprod6/2, dotprod7/2, dotprod8/2, dotprod9/2, dotprod10/2, dotprod11/2, dotprod12/2, dotprod13/2, dotprod14/2, dotprod15/2, dotprod16/2, dotprod17/2, dotprod18/2, dotprod19/2, dotprod20/2, dotprod21/2, dotprod22/2, dotprod23/2, dotprod24/2
  dotprod1/1 -> Mux/1
  "IW{1,1}(2,:)'"/1 -> dotprod2/1
  dotprod2/1 -> Mux/2
  "IW{1,1}(3,:)'"/1 -> dotprod3/1
  dotprod3/1 -> Mux/3
  "IW{1,1}(4,:)'"/1 -> dotprod4/1
  dotprod4/1 -> Mux/4
  "IW{1,1}(5,:)'"/1 -> dotprod5/1
  dotprod5/1 -> Mux/5
  "IW{1,1}(6,:)'"/1 -> dotprod6/1
  dotprod6/1 -> Mux/6
  "IW{1,1}(7,:)'"/1 -> dotprod7/1
  dotprod7/1 -> Mux/7
  "IW{1,1}(8,:)'"/1 -> dotprod8/1
  dotprod8/1 -> Mux/8
  "IW{1,1}(9,:)'"/1 -> dotprod9/1
  dotprod9/1 -> Mux/9
  "IW{1,1}(10,:)'"/1 -> dotprod10/1
  dotprod10/1 -> Mux/10
  "IW{1,1}(11,:)'"/1 -> dotprod11/1
  dotprod11/1 -> Mux/11
  "IW{1,1}(12,:)'"/1 -> dotprod12/1
  dotprod12/1 -> Mux/12
  "IW{1,1}(13,:)'"/1 -> dotprod13/1
  dotprod13/1 -> Mux/13
  "IW{1,1}(14,:)'"/1 -> dotprod14/1
  dotprod14/1 -> Mux/14
  "IW{1,1}(15,:)'"/1 -> dotprod15/1
  dotprod15/1 -> Mux/15
  "IW{1,1}(16,:)'"/1 -> dotprod16/1
  dotprod16/1 -> Mux/16
  "IW{1,1}(17,:)'"/1 -> dotprod17/1
  dotprod17/1 -> Mux/17
  "IW{1,1}(18,:)'"/1 -> dotprod18/1
  dotprod18/1 -> Mux/18
  "IW{1,1}(19,:)'"/1 -> dotprod19/1
  dotprod19/1 -> Mux/19
  "IW{1,1}(20,:)'"/1 -> dotprod20/1
  dotprod20/1 -> Mux/20
  "IW{1,1}(21,:)'"/1 -> dotprod21/1
  dotprod21/1 -> Mux/21
  "IW{1,1}(22,:)'"/1 -> dotprod22/1
  dotprod22/1 -> Mux/22
  "IW{1,1}(23,:)'"/1 -> dotprod23/1
  dotprod23/1 -> Mux/23
  "IW{1,1}(24,:)'"/1 -> dotprod24/1
  dotprod24/1 -> Mux/24
  Mux/1 -> "iz{1,1}"/1

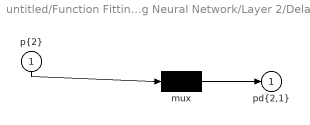
== system untitled/Function Fitting Neural Network/Layer 2/Delays 1 ==
  "p{2}" : Inport  PortDimensions=24
      mask Display: e = 0.06;c1 = [120 230 180]/255;c2 = ([120 230 180]+0)/(256+128);c3 = ([120 230 180]+128)/(256+128);patch([0 1 1 0],[0 0 1 1],c1);patch([0 1 1 1-e 1-e 0+e],[0 0 1 1-e 0+e 0+e],c2);patch([0 0 1 1-e 0+e 0+e],[0 1 1 1-e 1-e 0+e],c3);plot([0 1 1 0 0],[0 0 1 1 0]);
  mux : Mux  Inputs=1
      mask Display: e = 0.06;c1 = [120 150 230]/255;c2 = ([120 150 230]+0)/383;c3 = ([120 150 230]+128)/383;patch([0 1 1 0],[0 0 1 1],c1);patch([0 1 1 1-e 1-e 0+e],[0 0 1 1-e 0+e 0+e],c2);patch([0 0 1 1-e 0+e 0+e],[0 1 1 1-e 1-e 0+e],c3);plot([0 1 1 0 0],[0 0 1 1 0]);disp('Mux')
  "pd{2,1}" : Outport
      mask Display: e = 0.06;c1 = [120 230 180]/255;c2 = ([120 230 180]+0)/(256+128);c3 = ([120 230 180]+128)/(256+128);patch([0 1 1 0],[0 0 1 1],c1);patch([0 1 1 1-e 1-e 0+e],[0 0 1 1-e 0+e 0+e],c2);patch([0 0 1 1-e 0+e 0+e],[0 1 1 1-e 1-e 0+e],c3);plot([0 1 1 0 0],[0 0 1 1 0]);
  wires:
  "p{2}"/1 -> mux/1
  mux/1 -> "pd{2,1}"/1

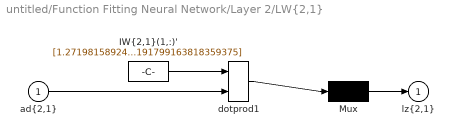
== system untitled/Function Fitting Neural Network/Layer 2/LW{2,1} ==
  "ad{2,1}" : Inport  PortDimensions=24
      mask Display: e = 0.06;c1 = [120 230 180]/255;c2 = ([120 230 180]+0)/(256+128);c3 = ([120 230 180]+128)/(256+128);patch([0 1 1 0],[0 0 1 1],c1);patch([0 1 1 1-e 1-e 0+e],[0 0 1 1-e 0+e 0+e],c2);patch([0 0 1 1-e 0+e 0+e],[0 1 1 1-e 1-e 0+e],c3);plot([0 1 1 0 0],[0 0 1 1 0]);
  "IW{2,1}(1,:)'" : Constant  Value=[1.2719815892408312674177750523085705935955047607421875;0.4681691700919550225279408550704829394817352294921875;-0.8113406966683502918868953202036209404468536376953125;-0.53002278385006296179682294678059406578540802001953125;1.025631233634657579756321865716017782688140869140625;-1.105278969524598142726290461723692715167999267578125;0.84120936477096763805860746288090012967586517333984375;-1.1335557282230503961528711442952044308185577392578125;0.78816121000741923285914936059270985424518585205078125;0.7130387429108122621101983895641751587390899658203125;-0.81825721543246776601421288432902656495571136474609375;-0.575106137247962667657930069253779947757720947265625;-0.92448372665336642217681628608261235058307647705078125;0.609117799968685869060891491244547069072723388671875;-0.63879343557323753355348117111134342849254608154296875;-0.5720240484049501361596412607468664646148681640625;-0.7748515759850758133353565426659770309925079345703125;-0.80093137624633625737402553568244911730289459228515625;0.57996883581627056702956224398803897202014923095703125;0.89262864406832653774159780368790961802005767822265625;0.8161959732106767173576145069091580808162689208984375;-0.53458598249496935839175648652599193155765533447265625;1.0145507811919112217680094545357860624790191650390625;0.8260609089397801252374620162299834191799163818359375]
      mask Display: e = 0.06;c1 = [120 150 230]/255;c2 = ([120 150 230]+0)/383;c3 = ([120 150 230]+128)/383;patch([0 1 1 0],[0 0 1 1],c1);patch([0 1 1 1-e 1-e 0+e],[0 0 1 1-e 0+e 0+e],c2);patch([0 0 1 1-e 0+e 0+e],[0 1 1 1-e 1-e 0+e],c3);plot([0 1 1 0 0],[0 0 1 1 0]);disp('weights');
  Mux : Mux  Inputs=1
      mask Display: e = 0.06;c1 = [120 150 230]/255;c2 = ([120 150 230]+0)/383;c3 = ([120 150 230]+128)/383;patch([0 1 1 0],[0 0 1 1],c1);patch([0 1 1 1-e 1-e 0+e],[0 0 1 1-e 0+e 0+e],c2);patch([0 0 1 1-e 0+e 0+e],[0 1 1 1-e 1-e 0+e],c3);plot([0 1 1 0 0],[0 0 1 1 0]);disp('Mux');
  dotprod1 : neural/Weight Functions/dotprod
  "lz{2,1}" : Outport
      mask Display: e = 0.06;c1 = [120 230 180]/255;c2 = ([120 230 180]+0)/(256+128);c3 = ([120 230 180]+128)/(256+128);patch([0 1 1 0],[0 0 1 1],c1);patch([0 1 1 1-e 1-e 0+e],[0 0 1 1-e 0+e 0+e],c2);patch([0 0 1 1-e 0+e 0+e],[0 1 1 1-e 1-e 0+e],c3);plot([0 1 1 0 0],[0 0 1 1 0]);
  wires:
  "IW{2,1}(1,:)'"/1 -> dotprod1/1
  "ad{2,1}"/1 -> dotprod1/2
  dotprod1/1 -> Mux/1
  Mux/1 -> "lz{2,1}"/1
